simulink model "CLIk"  (R2019a)
settings: Solver=VariableStepAuto  StartTime=0.0  StopTime=10  RelTol=1e-3
libraries: eeGeneralControl x1
settings Model: Creator=huic  LastModifiedBy=huic

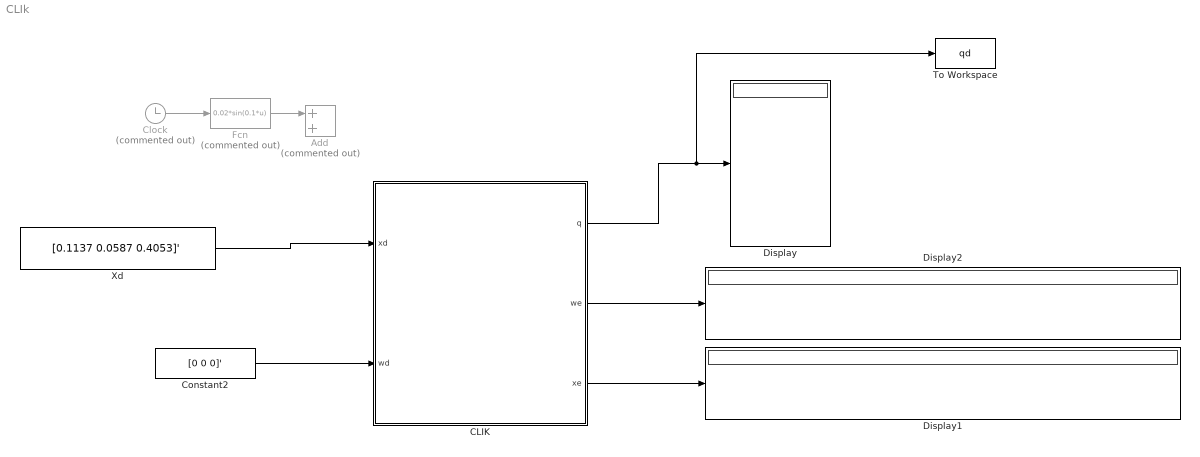
== system CLIk ==
  Add : Sum  Commented=on
  CLIK : Subsystem
  Clock : Clock  Commented=on
  Constant2 : Constant  Value=[0 0 0]'
  Display : Display
  Display1 : Display
  Display2 : Display
  Fcn : Fcn  Commented=on  Expr=0.02*sin(0.1*u)
  To Workspace : ToWorkspace  VariableName=qd  SaveFormat=Structure With Time  SampleTime=-1
  Xd : Constant  Value=[0.1137 0.0587 0.4053]'
  wires:
  Constant2/1 -> CLIK/2(wd)
  CLIK/1(q) -> To Workspace/1, Display/1
  CLIK/2(we) -> Display2/1
  CLIK/3(xe) -> Display1/1
  Clock/1 -> Fcn/1
  Fcn/1 -> Add/1
  Xd/1 -> CLIK/1(xd)

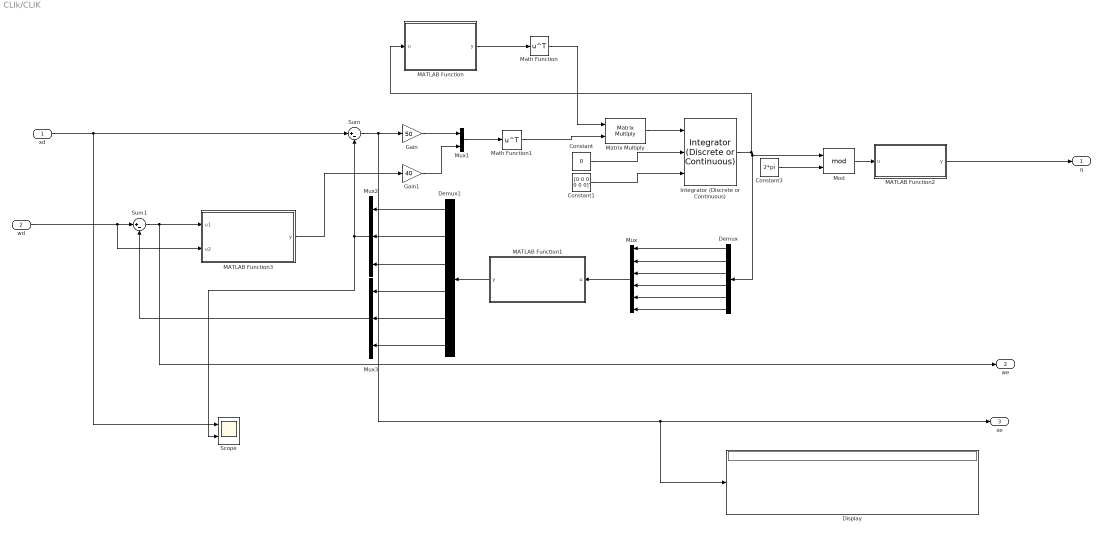
== system CLIk/CLIK ==
  xd : Inport
  wd : Inport  Port=2
  Constant : Constant  Value=0
  Constant1 : Constant  Value=[0 0 0 0 0 0]'
  Constant3 : Constant  Value=2*pi
  Demux : Demux  Outputs=[1 1 1 1 1 1]
  Demux1 : Demux  Outputs=[1 1 1 1 1 1]
  Display : Display
  Gain : Gain  Gain=50
  Gain1 : Gain  Gain=40
  Integrator (Discrete or Continuous) : eeGeneralControl/Integrator (Discrete or Continuous)  LabelModeActiveChoice=Continuous  ExternalReset=level  LimitType=Anti-windup  B=inf  A=-inf  Ts=0
      settings: SourceProductName=Simscape Electrical  SourceProductBaseCode=PS
  MATLAB Function : MATLAB Function  TreatAsAtomicUnit=on
  MATLAB Function1 : MATLAB Function  TreatAsAtomicUnit=on
  MATLAB Function2 : MATLAB Function  TreatAsAtomicUnit=on
  MATLAB Function3 : MATLAB Function  TreatAsAtomicUnit=on
  Math Function : Math  Operator=transpose  SaturateOnIntegerOverflow=on
  Math Function1 : Math  Operator=transpose  SaturateOnIntegerOverflow=on
  Matrix Multiply : Product  Multiplication=Matrix(*)
  Mod : Math  Operator=mod  SaturateOnIntegerOverflow=on
  Mux : Mux  Inputs=[1 1 1 1 1 1]
  Mux1 : Mux  Inputs=2
  Mux2 : Mux  Inputs=[1 1 1]
  Mux3 : Mux  Inputs=[1 1 1]
  Scope : Scope  NumInputPorts=2
  Sum : Sum  Inputs=|+-
  Sum1 : Sum  Inputs=|+-
  q : Outport
  we : Outport  Port=2
  xe : Outport  Port=3
  wires:
  MATLAB Function/1(y) -> Math Function/1
  Demux/2 -> Mux/2
  Gain/1 -> Mux1/1
  Integrator (Discrete or Continuous)/1 -> Demux/1, Mod/1, MATLAB Function/1(u)
  Math Function/1 -> Matrix Multiply/1
  Demux/5 -> Mux/5
  Mux/1 -> MATLAB Function1/1(u)
  MATLAB Function2/1(y) -> q/1
  Mux1/1 -> Math Function1/1
  Demux/4 -> Mux/4
  Demux1/5 -> Mux3/2
  MATLAB Function3/1(y) -> Gain1/1
  Demux/6 -> Mux/6
  wd/1 -> MATLAB Function3/2(u2), Sum1/1
  Demux/1 -> Mux/1
  Demux/3 -> Mux/3
  Matrix Multiply/1 -> Integrator (Discrete or Continuous)/1
  Sum/1 -> Display/1, xe/1, Gain/1
  Mux3/1 -> Sum1/2
  Constant3/1 -> Mod/2
  Mux2/1 -> Sum/2, Scope/2
  Demux1/4 -> Mux3/1
  Mod/1 -> MATLAB Function2/1(u)
  Demux1/1 -> Mux2/1
  Demux1/2 -> Mux2/2
  Gain1/1 -> Mux1/2
  MATLAB Function1/1(y) -> Demux1/1
  Math Function1/1 -> Matrix Multiply/2
  Demux1/3 -> Mux2/3
  Sum1/1 -> we/1, MATLAB Function3/1(u1)
  Constant1/1 -> Integrator (Discrete or Continuous)/3
  Demux1/6 -> Mux3/3
  xd/1 -> Scope/1, Sum/1
  Constant/1 -> Integrator (Discrete or Continuous)/2

== matlab function CLIk/CLIK/MATLAB Function1 ==
  data: u input; y output
function y = getpose(u)
a2=-0.2035;a3=-0.17442;d1=0.1205;d4=0.08009;
d5=0.08009;
q1=u(1);
q2=u(2);
q3=u(3);
q4=u(4);
q5=u(5);
q6=u(6);
%求运动学正解
T01 = [cos(q1) 0 sin(q1) 0;sin(q1) 0 -cos(q1) 0;0 1 0 d1;0 0 0 1];
T12 = [cos(q2) -sin(q2) 0 a2*cos(q2);sin(q2) cos(q2) 0 a2*sin(q2);0 0 1 0;0 0 0 1];
T23 = [cos(q3) -sin(q3) 0 a3*cos(q3);sin(q3) cos(q3) 0 a3*sin(q3);0 0 1 0;0 0 0 1];
T34 = [cos(q4) 0 sin(q4) 0;sin(q4) 0 -cos(q4) 0;0 1 0 d4;0 0 0 1];
T45 = [cos(q5) 0 -sin(q5)  0;sin(q5) 0 cos(q5) 0;0 -1 0 d5;0 0 0 1];
T56 = [cos(q6) -sin(q6) 0 0;sin(q6) cos(q6) 0 0;0 0 1 0;0 0 0 1];
T06 = T01*T12*T23*T34*T45*T56;

y1=T06(1:3,4);
y2=tform2eul(T06);
y=[y1;y2'];

== matlab function CLIk/CLIK/MATLAB Function ==
  data: u input; y output
function y = getjacob(u)
%标准型雅可比矩阵求解
a2=-0.2035;a3=-0.17442;d1=0.1205;d4=0.08009;
d5=0.08009;
q=u;
%求运动学正解
T01 = [cos(q(1)) 0 sin(q(1)) 0;sin(q(1)) 0 -cos(q(1)) 0;0 1 0 d1;0 0 0 1];
T12 = [cos(q(2)) -sin(q(2)) 0 a2*cos(q(2));sin(q(2)) cos(q(2)) 0 a2*sin(q(2));0 0 1 0;0 0 0 1];
T23 = [cos(q(3)) -sin(q(3)) 0 a3*cos(q(3));sin(q(3)) cos(q(3)) 0 a3*sin(q(3));0 0 1 0;0 0 0 1];
T34 = [cos(q(4)) 0 sin(q(4)) 0;sin(q(4)) 0 -cos(q(4)) 0;0 1 0 d4;0 0 0 1];
T45 = [cos(q(5)) 0 -sin(q(5))  0;sin(q(5)) 0 cos(q(5)) 0;0 -1 0 d5;0 0 0 1];
T56 = [cos(q(6)) -sin(q(6)) 0 0;sin(q(6)) cos(q(6)) 0 0;0 0 1 0;0 0 0 1];

k = [0; 0; 1];

%初始赋值
Jv = zeros(3, 6);
Jw = zeros(3, 6);
%获取每个关节原点与基座标的变换矩阵T01,T02...T06
% T{6}=zeros(4);
T=cell(6,1);
T{1}=T01;
T{2}=T{1}*T12;
T{3}=T{2}*T23;
T{4}=T{3}*T34;
T{5}=T{4}*T45;
T{6}=T{5}*T56;

%进行矢量积求解
for i = 1: 6
   if i == 1
       R = eye(3);
       p_im = T{6}(1: 3, 4);
   else
       R = T{i-1}(1: 3, 1: 3);
       p_im = T{6}(1: 3, 4) - T{i-1}(1: 3, 4);
   end
   
   zi_1 = R * k;
   Jv(:, i) = cross(zi_1, p_im);
   Jw(:, i) = zi_1;
end

% 组合
J = [Jv; Jw];
y=J;

== matlab function CLIk/CLIK/MATLAB Function2 ==
  data: u input; y output
function y = Joints_angle_Handle(u)
for i=1:6
    if(u(i) > pi)
        u(i) = u(i)-2*pi;
    elseif(u(i) < -pi)
        u(i) = u(i)+2*pi;
    end
end

y = u;

== matlab function CLIk/CLIK/MATLAB Function3 ==
  data: u1 input; y output; u2 input
function y = anglevelocity(u1,u2)
%u2为当前的欧拉角
%u1为欧拉角的变化量
tform=[cos(u2(2))*cos(u2(3)) -sin(u2(3)) 0;cos(u2(2))*sin(u2(3)) cos(u2(3)) 0;-sin(u2(2)) 0 1];
y=zeros(1,3);
dwxyz=tform*[u1(3);u1(2);u1(1)];
y(1)=dwxyz(1);
y(2)=dwxyz(2);
y(3)=dwxyz(3);
